simulink model "ESS_EV_Project_Simulink_Model"  (R2017a)
settings: Solver=FixedStepAuto  StartTime=0  StopTime=1369*75  RelTol=1e-3
values from neighbouring files (symbols this model uses):
  A = 2.2    [VehicleParameters.m]
  Cd = 0.28    [VehicleParameters.m]
  Cnom = 3.5    [VehicleParameters.m]
  Crr = 0.01    [VehicleParameters.m]
  g = 9.81    [VehicleParameters.m]
  Km = 1    [VehicleParameters.m]
  M = 1650    [VehicleParameters.m]
  Nchg = 0.85    [VehicleParameters.m]
  Ndrive = 0.98    [VehicleParameters.m]
  Ndsch = 0.9    [VehicleParameters.m]
  Nmotor = 0.95    [VehicleParameters.m]
  Np = round(Batt_cap_nominal*1000/(Ns*Vcell_nominal*Cnom))    [VehicleParameters.m]
  Ns = round(Vbatt_nominal/Vcell_nominal)    [VehicleParameters.m]
  Ntrans = 0.95    [VehicleParameters.m]
  rho = 1.2    [VehicleParameters.m]
  RP = 0.45    [VehicleParameters.m]
libraries: simulink x1, autolibshared x1
settings Model: Creator=JD  LastModifiedBy=JD

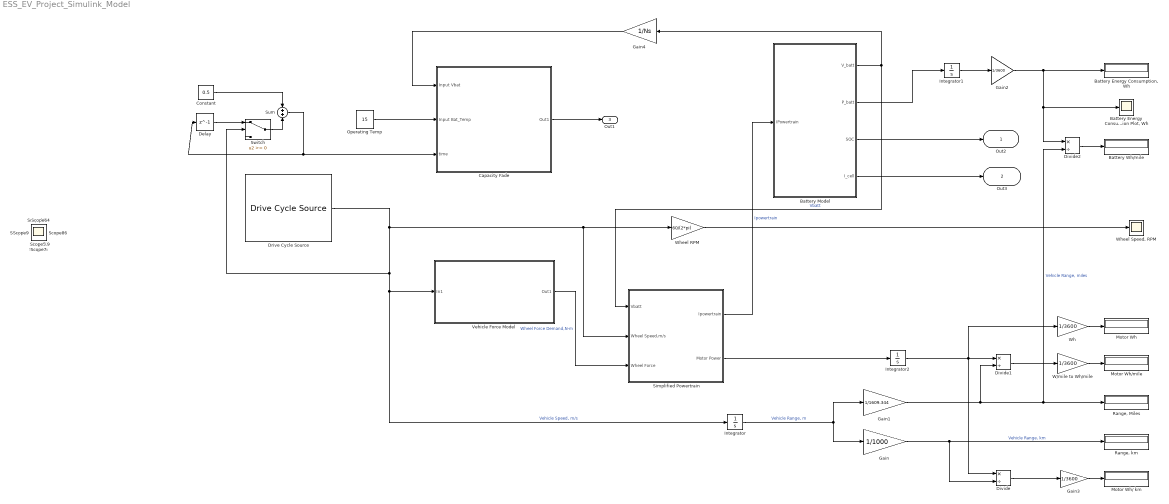
== system ESS_EV_Project_Simulink_Model ==
  "Battery Energy Consumption Plot, Wh" : Scope
  "Battery Energy Consumption, Wh" : Display
  Battery Model : Subsystem
  Battery Wh/mile : Display
  "Capacity Fade " : Subsystem
  Constant : Constant  Value=0.5
  Delay : Delay  DelayLength=1
  Divide : Product  Inputs=*/
  Divide1 : Product  Inputs=*/
  Divide2 : Product  Inputs=*/
  Drive Cycle Source : autolibshared/Drive Cycle Source  cycleVar=.mat, .xls, .xlsx or .txt file  fileVar=C:\Users\JD\MATLAB\Projects\ESS EV Project\Cycles\JC08 Cycle.xlsx  tfinal="1204  seconds, Cyclic"  cycleRepeat=on  outAccPort=off  t_wot1=5  xdot_woto=0  xdot_wot1=30  t_wot2=20  xdot_wot2=0  t_wotend=30  srcUnit=m/s  outUnit=m/s  srcAccUnit=m/s/s  outAccUnit=m/s^2  dt=0
      settings: SourceProductName=Powertrain Blockset  SourceProductBaseCode=PW
  Gain : Gain  Gain=1/1000
  Gain1 : Gain  Gain=1/1609.344
  Gain2 : Gain  Gain=1/3600
  Gain3 : Gain  Gain=1/3600
  Gain4 : Gain  Gain=1/Ns
  Integrator : Integrator
  Integrator1 : Integrator
  Integrator2 : Integrator
  Motor Wh : Display
  Motor Wh/ km : Display
  Motor Wh/mile : Display
  Operating Temp : Constant  Value=15
  "Range, Miles" : Display
  "Range, km" : Display
  Simplified Powertrain : Subsystem
  Sum : Sum
  Switch : Switch
  Vehicle Force Model : Subsystem
      mask Display: image('D:\Lecture Slides\MEEM 5275 - Energy Storage Systems\Project Resources\Report and Papers\Vehicle Forces.JPG');
  W/mile to Wh/mile : Gain  Gain=1/3600
  Wh : Gain  Gain=1/3600
  Wheel RPM : Gain  Gain=60/(2*pi)
  "Wheel Speed, RPM" : Scope
  Out2 : Outport  SignalName=SOC
  Out3 : Outport  Port=2  SignalName=I, cell
  Out1 : Outport  Port=3
  Scope{,1..19} (20 alike) : Scope
  wires:
  Drive Cycle Source/1 -> Simplified Powertrain/2(Wheel Speed,m/s), Wheel RPM/1, Integrator/1, Vehicle Force Model/1(In1), Switch/2  "Vehicle Speed, m/s"
  Vehicle Force Model/1(Out1) -> Simplified Powertrain/3(Wheel Force)  "Wheel Force Demand,N-m"
  Simplified Powertrain/1(Ipowertrain) -> Battery Model/1(IPowertrain)  "Ipowertrain"
  Integrator/1 -> Gain/1, Gain1/1  "Vehicle Range, m"
  Gain1/1 -> Divide2/2, "Range, Miles"/1, Divide1/2  "Vehicle Range, miles"
  Battery Model/1(V_batt) -> Gain4/1, Simplified Powertrain/1(Vbatt)  "Vbatt"
  Battery Model/4(I_cell) -> Out3/1
  Battery Model/3(SOC) -> Out2/1
  Battery Model/2(P_batt) -> Integrator1/1
  Integrator1/1 -> Gain2/1
  Gain2/1 -> "Battery Energy Consumption, Wh"/1, "Battery Energy Consumption Plot, Wh"/1, Divide2/1
  Integrator2/1 -> Wh/1, Divide/1, Divide1/1
  Divide1/1 -> W/mile to Wh/mile/1
  Simplified Powertrain/2(Motor Power) -> Integrator2/1
  W/mile to Wh/mile/1 -> Motor Wh/mile/1
  "Capacity Fade "/1(Out1) -> Out1/1
  Gain4/1 -> "Capacity Fade "/1(Input Vbat)
  Operating Temp/1 -> "Capacity Fade "/2(Input Bat_Temp)
  Switch/1 -> Sum/2
  Constant/1 -> Sum/1
  Sum/1 -> Delay/1, "Capacity Fade "/3(time)
  Delay/1 -> Switch/1
  Gain/1 -> Divide/2, "Range, km"/1  "Vehicle Range, km"
  Divide/1 -> Gain3/1
  Gain3/1 -> Motor Wh/ km/1
  Divide2/1 -> Battery Wh/mile/1
  Wh/1 -> Motor Wh/1
  Wheel RPM/1 -> "Wheel Speed, RPM"/1

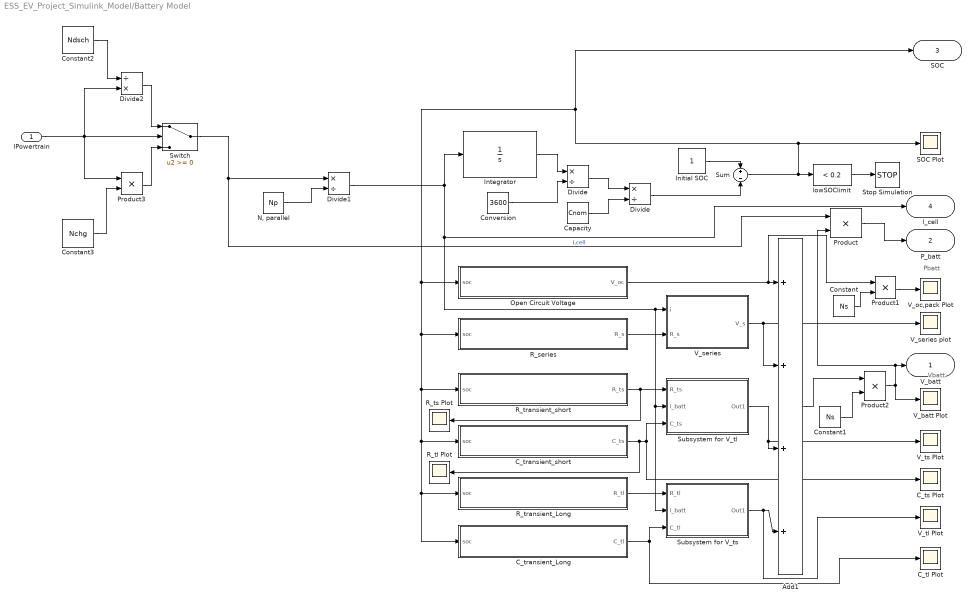
== system ESS_EV_Project_Simulink_Model/Battery Model ==
  note: Pbatt
  note: Vbatt
  IPowertrain : Inport
  Add1 : Sum  Inputs=++++
  C_tl Plot : Scope
  C_transient_Long : MATLAB Function  TreatAsAtomicUnit=on
  C_transient_short : MATLAB Function  TreatAsAtomicUnit=on
  C_ts Plot : Scope
  "Capacity " : Constant  Value=Cnom  SampleTime=1
  Constant : Constant  Value=Ns
  Constant1 : Constant  Value=Ns
  Constant2 : Constant  Value=Ndsch
  Constant3 : Constant  Value=Nchg
  Conversion : Constant  Value=3600  SampleTime=1
  Divide : Product  Inputs=*/
  "Divide " : Product  Inputs=*/
  Divide1 : Product  Inputs=*/
  Divide2 : Product  Inputs=/*
  Initial SOC : Constant  SampleTime=1
  Integrator : Integrator  InitialCondition=1
  "N, parallel" : Constant  Value=Np
  Open Circuit Voltage : MATLAB Function  TreatAsAtomicUnit=on
  Product{,1..3} (4 alike) : Product
  R_series : MATLAB Function  TreatAsAtomicUnit=on
  R_tl Plot : Scope
  R_transient_Long : MATLAB Function  TreatAsAtomicUnit=on
  R_transient_short : MATLAB Function  TreatAsAtomicUnit=on
  R_ts Plot : Scope
  "SOC Plot " : Scope
  Stop Simulation : Stop
  Subsystem for V_tl : Subsystem
  Subsystem for V_ts : Subsystem
  Sum : Sum  Inputs=+-
  Switch : Switch
  "V_batt Plot " : Scope
  "V_oc,pack Plot " : Scope
  V_series : MATLAB Function  TreatAsAtomicUnit=on
  "V_series plot " : Scope
  V_tl Plot : Scope
  "V_ts Plot " : Scope
  lowSOClimit : simulink/Logic and Bit Operations/Compare To Constant  relop=<  const=0.2  OutDataTypeStr=boolean
  V_batt : Outport
  P_batt : Outport  Port=2
  SOC : Outport  Port=3
  I_cell : Outport  Port=4
  wires:
  Divide/1 -> Sum/2
  C_transient_Long/1(C_tl) -> C_tl Plot/1, Subsystem for V_ts/3(C_tl)
  Subsystem for V_tl/1(Out1) -> "V_ts Plot "/1, Add1/3
  "Divide "/1 -> Divide/1
  Sum/1 -> lowSOClimit/1, "SOC Plot "/1, SOC/1, C_transient_Long/1(soc), R_transient_Long/1(soc), C_transient_short/1(soc), R_transient_short/1(soc), R_series/1(soc), Open Circuit Voltage/1(soc)
  Add1/1 -> Product2/1
  "Capacity "/1 -> Divide/2
  Conversion/1 -> "Divide "/2
  lowSOClimit/1 -> Stop Simulation/1
  C_transient_short/1(C_ts) -> Subsystem for V_tl/3(C_ts), C_ts Plot/1, R_tl Plot/1
  Open Circuit Voltage/1(V_oc) -> Product1/1, Add1/1
  R_transient_Long/1(R_tl) -> Subsystem for V_ts/1(R_tl)
  V_series/1(V_s) -> Add1/2, "V_series plot "/1
  R_transient_short/1(R_ts) -> Subsystem for V_tl/1(R_ts), R_ts Plot/1
  Initial SOC/1 -> Sum/1
  Product/1 -> P_batt/1
  Subsystem for V_ts/1(Out1) -> Add1/4, V_tl Plot/1
  Divide1/1 -> Subsystem for V_tl/2(i_batt), Subsystem for V_ts/2(i_batt), V_series/1(i), I_cell/1, Integrator/1  "I,cell"
  R_series/1(R_s) -> V_series/2(R_s)
  IPowertrain/1 -> Product3/1, Divide2/2, Switch/2
  "N, parallel"/1 -> Divide1/2
  Integrator/1 -> "Divide "/1
  Constant/1 -> Product1/2
  Constant1/1 -> Product2/2
  Product2/1 -> "V_batt Plot "/1, Product/2, V_batt/1
  Product1/1 -> "V_oc,pack Plot "/1
  Switch/1 -> Product/1, Divide1/1
  Constant2/1 -> Divide2/1
  Divide2/1 -> Switch/1
  Constant3/1 -> Product3/2
  Product3/1 -> Switch/3

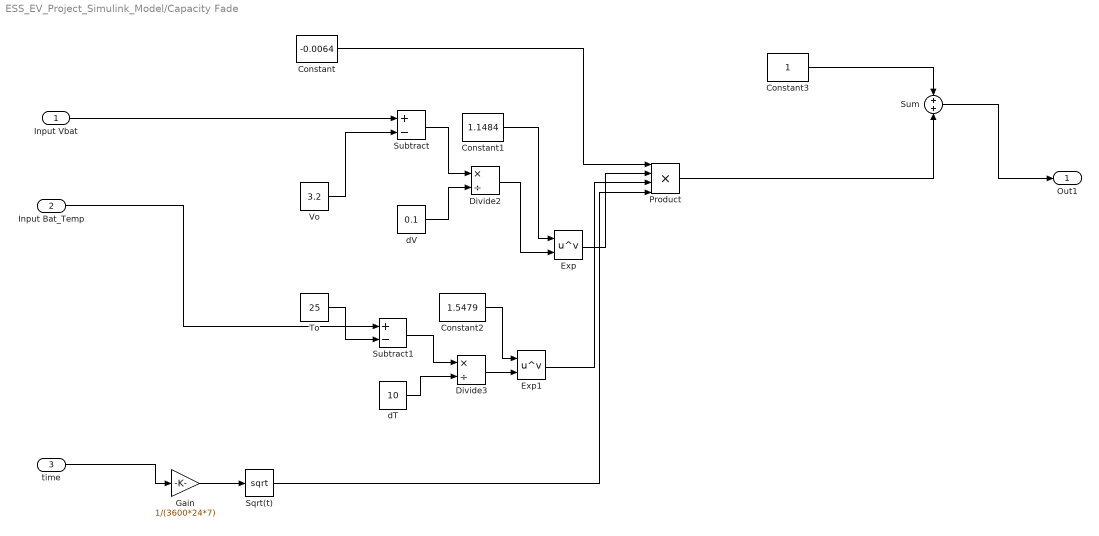
== system ESS_EV_Project_Simulink_Model/Capacity Fade  ==
  Input Vbat : Inport
  Input Bat_Temp : Inport  Port=2
  time : Inport  Port=3
  Constant : Constant  Value=-0.0064
  Constant1 : Constant  Value=1.1484
  Constant2 : Constant  Value=1.5479
  Constant3 : Constant
  Divide2 : Product  Inputs=*/
  Divide3 : Product  Inputs=*/
  Exp : Math  Operator=pow  SaturateOnIntegerOverflow=on
  Exp1 : Math  Operator=pow  SaturateOnIntegerOverflow=on
  Gain : Gain  Gain=1/(3600*24*7)
  Product : Product  Inputs=4
  Sqrt(t) : Sqrt  SaturateOnIntegerOverflow=on
  Subtract : Sum  Inputs=+-
  Subtract1 : Sum  Inputs=+-
  Sum : Sum
  To : Constant  Value=25
  Vo : Constant  Value=3.2
  dT : Constant  Value=10
  dV : Constant  Value=0.1
  Out1 : Outport
  wires:
  dT/1 -> Divide3/2
  Constant3/1 -> Sum/1
  Input Vbat/1 -> Subtract/1
  Divide3/1 -> Exp1/2
  dV/1 -> Divide2/2
  Input Bat_Temp/1 -> Subtract1/1
  Constant/1 -> Product/1
  Divide2/1 -> Exp/2
  Sum/1 -> Out1/1
  Product/1 -> Sum/2
  Exp/1 -> Product/2
  To/1 -> Subtract1/2
  Exp1/1 -> Product/3
  Constant1/1 -> Exp/1
  time/1 -> Gain/1
  Subtract1/1 -> Divide3/1
  Subtract/1 -> Divide2/1
  Sqrt(t)/1 -> Product/4
  Constant2/1 -> Exp1/1
  Vo/1 -> Subtract/2
  Gain/1 -> Sqrt(t)/1

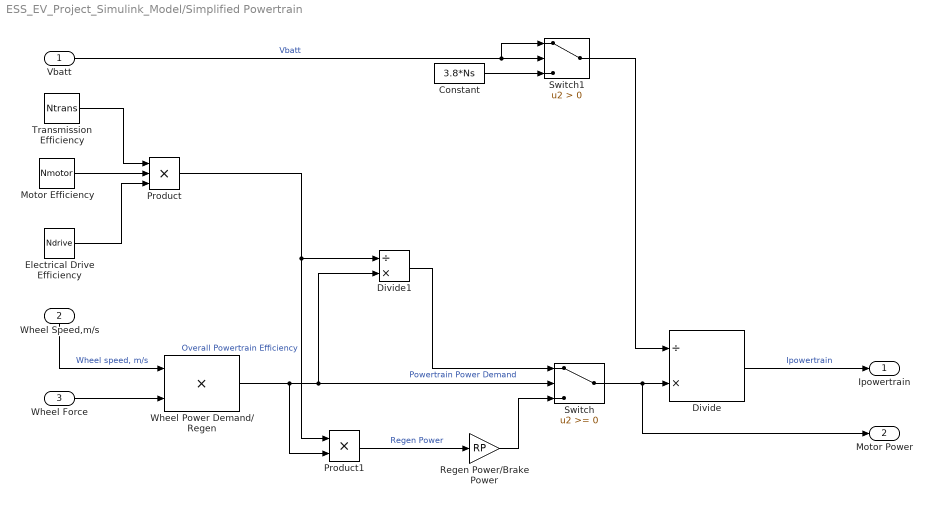
== system ESS_EV_Project_Simulink_Model/Simplified Powertrain ==
  Vbatt : Inport  SampleTime=10
  Wheel Speed,m/s : Inport  Port=2
  Wheel Force : Inport  Port=3
  Constant : Constant  Value=3.8*Ns
  Divide : Product  Inputs=/*
  Divide1 : Product  Inputs=/*
  Electrical Drive Efficiency : Constant  Value=Ndrive
  Motor Efficiency : Constant  Value=Nmotor
  Product : Product  Inputs=3
  Product1 : Product
  Regen Power/Brake Power : Gain  Gain=RP
  Switch : Switch
  Switch1 : Switch  Criteria=u2 > Threshold  OutDataTypeStr=double  RndMeth=Convergent
      settings: LockScale=on
  Transmission Efficiency : Constant  Value=Ntrans
  "Wheel Power Demand/ Regen " : Product
  Ipowertrain : Outport
  Motor Power : Outport  Port=2
  wires:
  Divide/1 -> Ipowertrain/1  "Ipowertrain"
  Wheel Force/1 -> "Wheel Power Demand/ Regen "/2
  Wheel Speed,m/s/1 -> "Wheel Power Demand/ Regen "/1  "Wheel speed, m/s"
  Transmission Efficiency/1 -> Product/1
  Motor Efficiency/1 -> Product/2
  Electrical Drive Efficiency/1 -> Product/3
  Product/1 -> Divide1/1, Product1/1  "Overall Powertrain Efficiency"
  "Wheel Power Demand/ Regen "/1 -> Divide1/2, Switch/2, Product1/2
  Divide1/1 -> Switch/1  "Powertrain Power Demand"
  Switch/1 -> Motor Power/1, Divide/2
  Product1/1 -> Regen Power/Brake Power/1  "Regen Power"
  Regen Power/Brake Power/1 -> Switch/3
  Vbatt/1 -> Switch1/1, Switch1/2  "Vbatt"
  Constant/1 -> Switch1/3
  Switch1/1 -> Divide/1

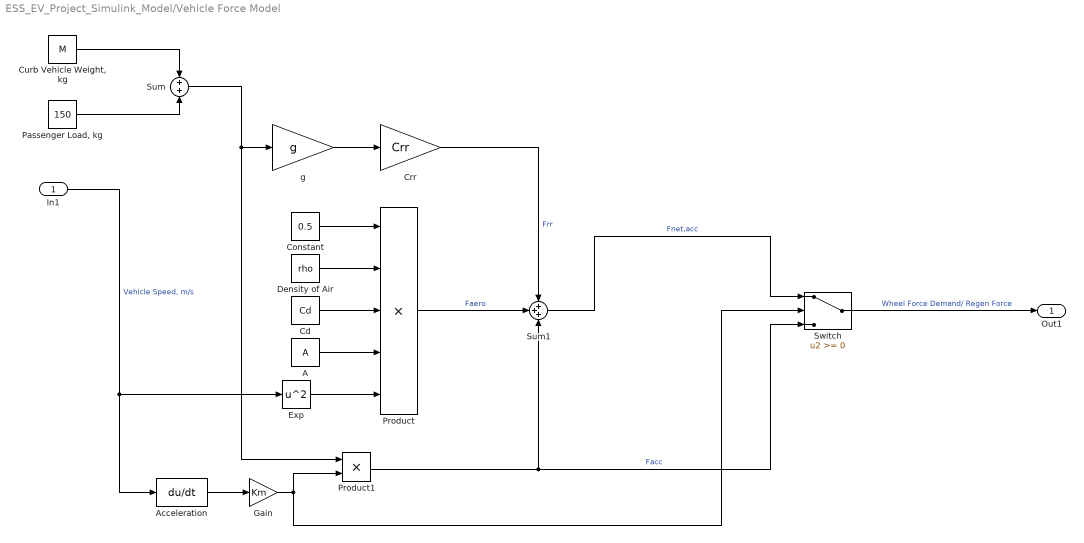
== system ESS_EV_Project_Simulink_Model/Vehicle Force Model ==
  In1 : Inport
  A : Constant  Value=A
  Acceleration : Derivative  CoefficientInTFapproximation=1
  Cd : Constant  Value=Cd
  Constant : Constant  Value=0.5
  Crr : Gain  Gain=Crr
  "Curb Vehicle Weight, kg" : Constant  Value=M
  Density of Air : Constant  Value=rho
  Exp : Math  Operator=square  SaturateOnIntegerOverflow=on
  Gain : Gain  Gain=Km
  "Passenger Load, kg" : Constant  Value=150
  Product : Product  Inputs=5
  Product1 : Product
  Sum : Sum
  Sum1 : Sum  Inputs=+++
  Switch : Switch
  g : Gain  Gain=g
  Out1 : Outport
  wires:
  g/1 -> Crr/1
  Exp/1 -> Product/5
  Product/1 -> Sum1/2  "Faero"
  Density of Air/1 -> Product/2
  Cd/1 -> Product/3
  A/1 -> Product/4
  Constant/1 -> Product/1
  Product1/1 -> Switch/3, Sum1/3  "Facc"
  Sum1/1 -> Switch/1  "Fnet,acc"
  Crr/1 -> Sum1/1  "Frr"
  In1/1 -> Exp/1, Acceleration/1  "Vehicle Speed, m/s"
  Acceleration/1 -> Gain/1
  Switch/1 -> Out1/1  "Wheel Force Demand/ Regen Force"
  "Passenger Load, kg"/1 -> Sum/2
  Sum/1 -> Product1/1, g/1
  "Curb Vehicle Weight, kg"/1 -> Sum/1
  Gain/1 -> Switch/2, Product1/2

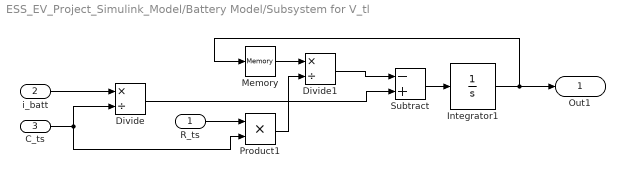
== system ESS_EV_Project_Simulink_Model/Battery Model/Subsystem for V_tl ==
  R_ts : Inport
  i_batt : Inport  Port=2
  C_ts : Inport  Port=3
  Divide : Product  Inputs=*/
  Divide1 : Product  Inputs=*/
  Integrator1 : Integrator
  Memory : Memory
  Product1 : Product
  "Subtract " : Sum  Inputs=-+
  Out1 : Outport
  wires:
  Divide/1 -> "Subtract "/2
  Memory/1 -> Divide1/1
  Divide1/1 -> "Subtract "/1
  R_ts/1 -> Product1/1
  Product1/1 -> Divide1/2
  Integrator1/1 -> Out1/1, Memory/1
  i_batt/1 -> Divide/1
  C_ts/1 -> Product1/2, Divide/2
  "Subtract "/1 -> Integrator1/1

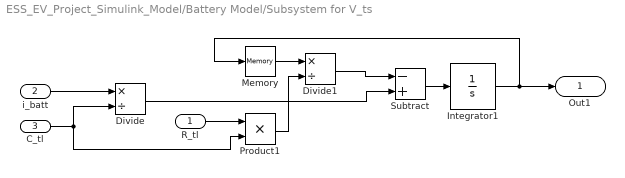
== system ESS_EV_Project_Simulink_Model/Battery Model/Subsystem for V_ts ==
  R_tl : Inport
  i_batt : Inport  Port=2
  C_tl : Inport  Port=3
  Divide : Product  Inputs=*/
  Divide1 : Product  Inputs=*/
  Integrator1 : Integrator
  Memory : Memory
  Product1 : Product
  "Subtract " : Sum  Inputs=-+
  Out1 : Outport
  wires:
  i_batt/1 -> Divide/1
  Product1/1 -> Divide1/2
  Integrator1/1 -> Out1/1, Memory/1
  C_tl/1 -> Product1/2, Divide/2
  Memory/1 -> Divide1/1
  R_tl/1 -> Product1/1
  Divide/1 -> "Subtract "/2
  "Subtract "/1 -> Integrator1/1
  Divide1/1 -> "Subtract "/1

== matlab function ESS_EV_Project_Simulink_Model/Battery Model/R_series ==
  data: soc input; R_s output
function R_s = fcn(soc)

R_s = 0.1562*exp(-24.37*soc)+0.07446;

== matlab function ESS_EV_Project_Simulink_Model/Battery Model/Open Circuit Voltage ==
  data: soc input; V_oc output
function V_oc = fcn(soc)
%#codegen

%syms soc
V_oc = -1.031*exp(-35*soc) + 3.685 + 0.2156*soc - 0.1178*soc^2 + 0.3201*soc^3;
%soc = 0.0:0.01:1.0;
%SOC = meshgrid(soc);
%plot(SOC(1,:),subs(V_oc,soc(1,:)));

== matlab function ESS_EV_Project_Simulink_Model/Battery Model/R_transient_short ==
  data: soc input; R_ts output
function R_ts = fcn(soc)

R_ts = 0.3208*exp(-29.14*soc)+0.04669;

== matlab function ESS_EV_Project_Simulink_Model/Battery Model/C_transient_short ==
  data: soc input; C_ts output
function C_ts = fcn(soc)

C_ts = -752.9*exp(-13.51*soc)+703.6;

== matlab function ESS_EV_Project_Simulink_Model/Battery Model/R_transient_Long ==
  data: soc input; R_tl output
function R_tl = fcn(soc)

R_tl = 6.603*exp(-155.2*soc)+0.04984;

== matlab function ESS_EV_Project_Simulink_Model/Battery Model/C_transient_Long ==
  data: soc input; C_tl output
function C_tl = fcn(soc)

C_tl = -6065*exp(-27.12*soc)+4475;

== matlab function ESS_EV_Project_Simulink_Model/Battery Model/V_series ==
  data: i input; V_s output; R_s input
function V_s = fcn(i,R_s)

V_s = i*R_s;
